simulink model "test_dram_sim"  (Simulink 6.2)
settings: Solver=ode45  StartTime=0.0  StopTime=14000  RelTol=1e-3
undefined symbols (not defined in the file): ant_bits
libraries: xbsIndex_r3 x353, xps_library x9, casper_library x8
(part 1 of 2)
settings Model: LastModifiedBy=humbert
settings DebuggingCC: SolverPrmCheckMsg=warning

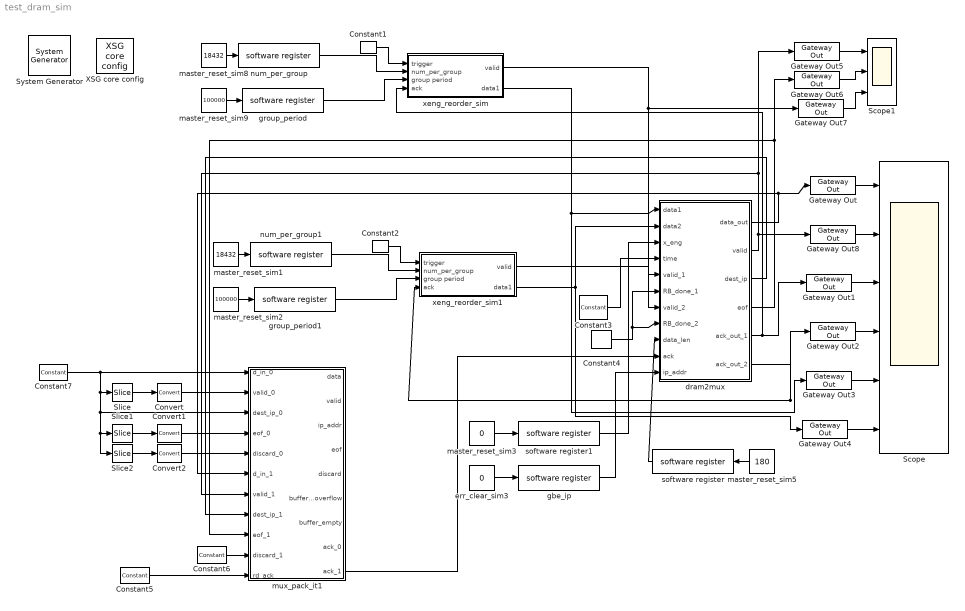
== system test_dram_sim ==
  " System Generator" : xbsIndex_r3/ System Generator  Tag=genX  xilinxfamily=Virtex2  part=xc2v1000  speed=-4  package=bg575  synthesis_tool=XST  directory=./netlist  testbench=off  simulink_period=1  sysclk_period=100  incr_netlist=off  trim_vbits=Everywhere in SubSystem  dbl_ovrd=According to Block Masks  core_generation=According to Block Masks  run_coregen=off  deprecated_control=off  eval_field=0
      settings: AttributesFormatString=System\nGenerator
  Constant1 : xbsIndex_r3/Constant  const=1  equ=P=C  arith_type=Boolean  n_bits=1  bin_pt=0  opselect=C  inp2=PCIN>>17  opr=+  inp1=P  carry=CIN  iostate=0  explicit_period=on  period=1  dbl_ovrd=off
  Constant2 : xbsIndex_r3/Constant  const=1  equ=P=C  arith_type=Boolean  n_bits=1  bin_pt=0  opselect=C  inp2=PCIN>>17  opr=+  inp1=P  carry=CIN  iostate=0  explicit_period=on  period=1  dbl_ovrd=off
  Constant3 : xbsIndex_r3/Constant  const=300  equ=P=C  arith_type=Unsigned  n_bits=64  bin_pt=0  opselect=C  inp2=PCIN>>17  opr=+  inp1=P  carry=CIN  iostate=0  explicit_period=on  period=1  dbl_ovrd=off
  Constant4 : xbsIndex_r3/Constant  const=0  equ=P=C  arith_type=Unsigned  n_bits=1  bin_pt=0  opselect=C  inp2=PCIN>>17  opr=+  inp1=P  carry=CIN  iostate=0  explicit_period=on  period=1  dbl_ovrd=off
  Constant5 : xbsIndex_r3/Constant  const=1  equ=P=C  arith_type=Boolean  n_bits=1  bin_pt=0  opselect=C  inp2=PCIN>>17  opr=+  inp1=P  carry=CIN  iostate=0  explicit_period=on  period=1  dbl_ovrd=off
  Constant6 : xbsIndex_r3/Constant  const=0  equ=P=C  arith_type=Boolean  n_bits=32  bin_pt=0  opselect=C  inp2=PCIN>>17  opr=+  inp1=P  carry=CIN  iostate=0  explicit_period=on  period=1  dbl_ovrd=off
  Constant7 : xbsIndex_r3/Constant  const=0  equ=P=C  arith_type=Unsigned  n_bits=32  bin_pt=0  opselect=C  inp2=PCIN>>17  opr=+  inp1=P  carry=CIN  iostate=0  explicit_period=on  period=1  dbl_ovrd=off
  Convert : xbsIndex_r3/Convert  arith_type=Boolean  n_bits=8  bin_pt=6  quantization=Truncate  overflow=Wrap  latency=0  explicit_period=off  period=1  dbl_ovrd=off  show_param=off  inserted_by_tool=off  pipeline=off
      settings: xl_area=[0, 0, 0, 0, 0, 0, 0]
  Convert1 : xbsIndex_r3/Convert  arith_type=Boolean  n_bits=8  bin_pt=6  quantization=Truncate  overflow=Wrap  latency=0  explicit_period=off  period=1  dbl_ovrd=off  show_param=off  inserted_by_tool=off  pipeline=off
      settings: xl_area=[0, 0, 0, 0, 0, 0, 0]
  Convert2 : xbsIndex_r3/Convert  arith_type=Boolean  n_bits=8  bin_pt=6  quantization=Truncate  overflow=Wrap  latency=0  explicit_period=off  period=1  dbl_ovrd=off  show_param=off  inserted_by_tool=off  pipeline=off
      settings: xl_area=[0, 0, 0, 0, 0, 0, 0]
  Gateway Out{,1..8} (9 alike) : xbsIndex_r3/Gateway Out  output_type=Double  nbits=8  bin_pt=6  arith_type=Boolean  quantization=Truncate  overflow=Wrap  hdl_port=on  timing_constraint=None  locs_specified=off  LOCs={}  needs_fixed_name=off  show_param=off
      settings: xl_area=[0, 0, 0, 0, 0, 0, 0]
  Scope : Scope  NumInputPorts=6
      settings: YMin=0~0~0~0~965~900  YMax=1000~1~1~1~995~930  MaxDataPoints=10000
  Scope1 : Scope  NumInputPorts=3
      settings: YMin=-5~-5~-5  YMax=5~5~5  SaveName=ScopeData6  MaxDataPoints=10000
  Slice : xbsIndex_r3/Slice  mode=Lower Bit Location + Width  nbits=1  bit1=0  base1=MSB of Input  bit0=0  base0=LSB of Input  boolean_output=off  explicit_period=off  period=1  dbl_ovrd=off
  Slice1 : xbsIndex_r3/Slice  mode=Lower Bit Location + Width  nbits=1  bit1=0  base1=MSB of Input  bit0=0  base0=LSB of Input  boolean_output=off  explicit_period=off  period=1  dbl_ovrd=off
  Slice2 : xbsIndex_r3/Slice  mode=Lower Bit Location + Width  nbits=1  bit1=0  base1=MSB of Input  bit0=0  base0=LSB of Input  boolean_output=off  explicit_period=off  period=1  dbl_ovrd=off
  XSG core config : xps_library/XSG core config  Tag=xps:xsg  hw_sys=BEE2_usr  ibob_linux=off  clk_src=sys_clk2x  gpio_clk_io_group=iBOB:sma  gpio_clk_bit_index=0  clk_rate=205  sample_period=1  synthesis_tool=XST  mpc_type=powerpc405
  dram2mux : Subsystem
  err_clear_sim3 : Constant  Value=0
  gbe_ip : xps_library/software register  Tag=xps:sw_reg  io_dir=From Processor  arith_type=Unsigned  bitwidth=32  bin_pt=0  sample_period=1  gw_name=test_dram_sim_gbe_ip_user_data_out
  group_period : xps_library/software register  Tag=xps:sw_reg  io_dir=From Processor  arith_type=Unsigned  bitwidth=32  bin_pt=0  sample_period=1  gw_name=test_dram_sim_group_period_user_data_out
  group_period1 : xps_library/software register  Tag=xps:sw_reg  io_dir=From Processor  arith_type=Unsigned  bitwidth=32  bin_pt=0  sample_period=1  gw_name=test_dram_sim_group_period1_user_data_out
  master_reset_sim1 : Constant  Value=18432
  master_reset_sim2 : Constant  Value=100000
  master_reset_sim3 : Constant  Value=0
  master_reset_sim5 : Constant  Orientation=left  Value=180
  master_reset_sim8 : Constant  Value=18432
  master_reset_sim9 : Constant  Value=100000
  mux_pack_it1 : Subsystem  mask(mux_packets){max_packet_size_0=1500, min_packet_size_0=50, max_packet_size_1=1500, min_packet_size_1=50}
      mask prompts: max_packet_size_0 "Input 0: Maximum single packet size (words)"; min_packet_size_0 "Input 0: Minimum single packet size (words)"; max_packet_size_1 "Input 1: Maximum single packet size (words)"; min_packet_size_1 "Input 1: Minimum single packet size (words)"
      mask help: This block allows you to mux together two data streams to be sent to the 10GbE core
  num_per_group : xps_library/software register  Tag=xps:sw_reg  io_dir=From Processor  arith_type=Unsigned  bitwidth=32  bin_pt=0  sample_period=1  gw_name=test_dram_sim_num_per_group_user_data_out
  num_per_group1 : xps_library/software register  Tag=xps:sw_reg  io_dir=From Processor  arith_type=Unsigned  bitwidth=32  bin_pt=0  sample_period=1  gw_name=test_dram_sim_num_per_group1_user_data_out
  software register : xps_library/software register  Tag=xps:sw_reg  Orientation=left  io_dir=From Processor  arith_type=Unsigned  bitwidth=32  bin_pt=0  sample_period=1  gw_name=test_dram_sim_software_register_user_data_out
  software register1 : xps_library/software register  Tag=xps:sw_reg  io_dir=From Processor  arith_type=Unsigned  bitwidth=32  bin_pt=0  sample_period=1  gw_name=test_dram_sim_software_register1_user_data_out
  xeng_reorder_sim : Subsystem
  xeng_reorder_sim1 : Subsystem
  wires:
  num_per_group/1 -> xeng_reorder_sim/2(num_per_group)
  master_reset_sim8/1 -> num_per_group/1
  group_period/1 -> xeng_reorder_sim/3(group period)
  master_reset_sim9/1 -> group_period/1
  Constant1/1 -> xeng_reorder_sim/1(trigger)
  num_per_group1/1 -> xeng_reorder_sim1/2(num_per_group)
  master_reset_sim1/1 -> num_per_group1/1
  group_period1/1 -> xeng_reorder_sim1/3(group period)
  master_reset_sim2/1 -> group_period1/1
  Constant2/1 -> xeng_reorder_sim1/1(trigger)
  xeng_reorder_sim/2(data1) -> Gateway Out3/1, dram2mux/1(data1)
  xeng_reorder_sim1/2(data1) -> Gateway Out4/1, dram2mux/2(data2)
  xeng_reorder_sim/1(valid) -> dram2mux/5(valid_1), Gateway Out7/1
  xeng_reorder_sim1/1(valid) -> dram2mux/7(valid_2)
  master_reset_sim3/1 -> software register1/1
  software register1/1 -> dram2mux/3(x_eng)
  Constant3/1 -> dram2mux/4(time)
  Constant4/1 -> dram2mux/8(RB_done_2), dram2mux/6(RB_done_1)
  master_reset_sim5/1 -> software register/1
  software register/1 -> dram2mux/9(data_len)
  err_clear_sim3/1 -> gbe_ip/1
  gbe_ip/1 -> dram2mux/11(ip_addr)
  dram2mux/5(ack_out_1) -> xeng_reorder_sim/4(ack), Gateway Out1/1
  dram2mux/6(ack_out_2) -> xeng_reorder_sim1/4(ack), Gateway Out2/1
  Gateway Out/1 -> Scope/1
  dram2mux/1(data_out) -> Gateway Out/1, mux_pack_it1/6(d_in_1)
  dram2mux/2(valid) -> mux_pack_it1/7(valid_1), Gateway Out5/1, Gateway Out8/1
  dram2mux/3(dest_ip) -> mux_pack_it1/8(dest_ip_1)
  Constant5/1 -> mux_pack_it1/11(rd_ack)
  Constant6/1 -> mux_pack_it1/10(discard_1)
  mux_pack_it1/9(ack_1) -> dram2mux/10(ack)
  Constant7/1 -> mux_pack_it1/1(d_in_0), mux_pack_it1/3(dest_ip_0), Slice1/1, Slice2/1, Slice/1
  Slice/1 -> Convert/1
  Convert/1 -> mux_pack_it1/2(valid_0)
  Slice1/1 -> Convert1/1
  Slice2/1 -> Convert2/1
  Convert1/1 -> mux_pack_it1/4(eof_0)
  Convert2/1 -> mux_pack_it1/5(discard_0)
  Gateway Out5/1 -> Scope1/1
  Gateway Out6/1 -> Scope1/2
  dram2mux/4(eof) -> mux_pack_it1/9(eof_1), Gateway Out6/1
  Gateway Out7/1 -> Scope1/3
  Gateway Out4/1 -> Scope/6
  Gateway Out3/1 -> Scope/5
  Gateway Out2/1 -> Scope/4
  Gateway Out1/1 -> Scope/3
  Gateway Out8/1 -> Scope/2

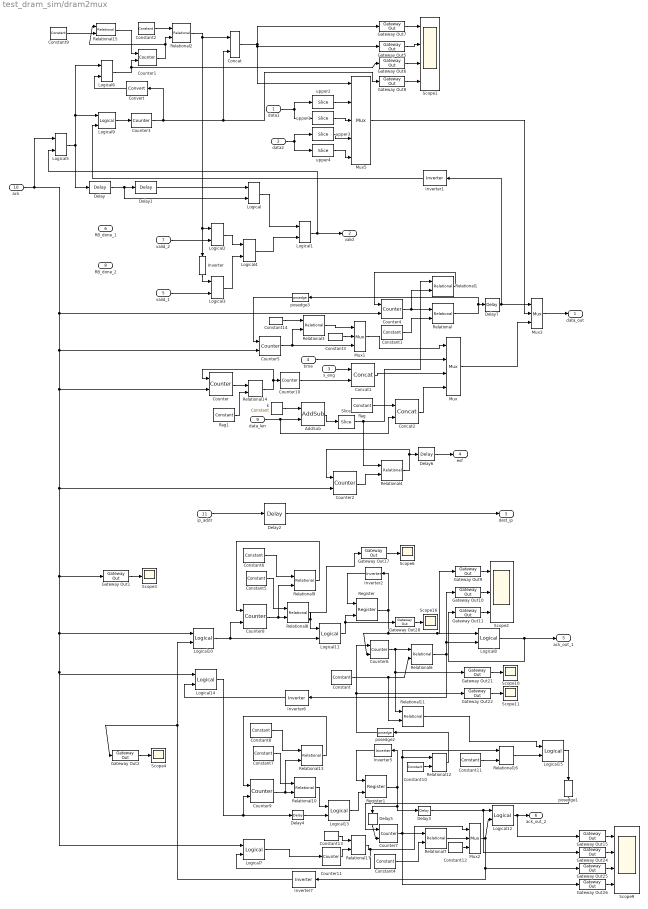
== system test_dram_sim/dram2mux ==
  data1 : Inport  Port=1  LatchInput=off
  data2 : Inport  Port=2  LatchInput=off
  x_eng : Inport  Port=3  LatchInput=off
  time : Inport  Port=4  LatchInput=off
  valid_1 : Inport  Port=5  LatchInput=off
  RB_done_1 : Inport  Port=6  LatchInput=off
  valid_2 : Inport  Port=7  LatchInput=off
  RB_done_2 : Inport  Port=8  LatchInput=off
  data_len : Inport  Port=9  LatchInput=off
  ack : Inport  Port=10  LatchInput=off
  ip_addr : Inport  Port=11  LatchInput=off
  AddSub : xbsIndex_r3/AddSub  mode=Addition  precision=Full  arith_type=Unsigned  n_bits=8  bin_pt=2  quantization=Truncate  overflow=Wrap  latency=0  explicit_period=off  period=1  use_carryin=off  use_carryout=off  en=off  dbl_ovrd=off  show_param=off  use_core=on  pipeline=off  use_rpm=on  gen_core=off
      settings: xl_area=[0, 0, 0, 0, 0, 0, 0]
  Concat : xbsIndex_r3/Concat  num_inputs=2  explicit_period=off  period=1  dbl_ovrd=off
  Concat1 : xbsIndex_r3/Concat  num_inputs=2  explicit_period=off  period=1  dbl_ovrd=off
  Concat2 : xbsIndex_r3/Concat  num_inputs=2  explicit_period=off  period=1  dbl_ovrd=off
  Constant : xbsIndex_r3/Constant  const=269  equ=P=C  arith_type=Unsigned  n_bits=9  bin_pt=0  opselect=C  inp2=PCIN>>17  opr=+  inp1=P  carry=CIN  iostate=0  explicit_period=on  period=1  dbl_ovrd=off
  Constant1 : xbsIndex_r3/Constant  const=3  equ=P=C  arith_type=Unsigned  n_bits=16  bin_pt=0  opselect=C  inp2=PCIN>>17  opr=+  inp1=P  carry=CIN  iostate=0  explicit_period=on  period=1  dbl_ovrd=off
  Constant10 : xbsIndex_r3/Constant  const=269  equ=P=C  arith_type=Unsigned  n_bits=9  bin_pt=0  opselect=C  inp2=PCIN>>17  opr=+  inp1=P  carry=CIN  iostate=0  explicit_period=on  period=1  dbl_ovrd=off
  Constant11 : xbsIndex_r3/Constant  const=271  equ=P=C  arith_type=Unsigned  n_bits=9  bin_pt=0  opselect=C  inp2=PCIN>>17  opr=+  inp1=P  carry=CIN  iostate=0  explicit_period=on  period=1  dbl_ovrd=off
  Constant12 : xbsIndex_r3/Constant  const=0  equ=P=C  arith_type=Boolean  n_bits=1  bin_pt=0  opselect=C  inp2=PCIN>>17  opr=+  inp1=P  carry=CIN  iostate=0  explicit_period=on  period=1  dbl_ovrd=off
  Constant13 : xbsIndex_r3/Constant  const=183  equ=P=C  arith_type=Unsigned  n_bits=10  bin_pt=0  opselect=C  inp2=PCIN>>17  opr=+  inp1=P  carry=CIN  iostate=0  explicit_period=on  period=1  dbl_ovrd=off
  Constant14 : xbsIndex_r3/Constant  const=2  equ=P=C  arith_type=Unsigned  n_bits=2  bin_pt=0  opselect=C  inp2=PCIN>>17  opr=+  inp1=P  carry=CIN  iostate=0  explicit_period=on  period=1  dbl_ovrd=off
  Constant2 : xbsIndex_r3/Constant  const=90  equ=P=C  arith_type=Unsigned  n_bits=8  bin_pt=0  opselect=C  inp2=PCIN>>17  opr=+  inp1=P  carry=CIN  iostate=0  explicit_period=on  period=1  dbl_ovrd=off
  Constant3 : xbsIndex_r3/Constant  const=0  equ=P=C  arith_type=Unsigned  n_bits=1  bin_pt=0  opselect=C  inp2=PCIN>>17  opr=+  inp1=P  carry=CIN  iostate=0  explicit_period=on  period=1  dbl_ovrd=off
  Constant4 : xbsIndex_r3/Constant  const=269  equ=P=C  arith_type=Unsigned  n_bits=9  bin_pt=0  opselect=C  inp2=PCIN>>17  opr=+  inp1=P  carry=CIN  iostate=0  explicit_period=on  period=1  dbl_ovrd=off
  Constant5 : xbsIndex_r3/Constant  const=3  equ=P=C  arith_type=Unsigned  n_bits=2  bin_pt=0  opselect=C  inp2=PCIN>>17  opr=+  inp1=P  carry=CIN  iostate=0  explicit_period=on  period=1  dbl_ovrd=off
  Constant6 : xbsIndex_r3/Constant  const=183  equ=P=C  arith_type=Unsigned  n_bits=8  bin_pt=0  opselect=C  inp2=PCIN>>17  opr=+  inp1=P  carry=CIN  iostate=0  explicit_period=on  period=1  dbl_ovrd=off
  Constant7 : xbsIndex_r3/Constant  const=3  equ=P=C  arith_type=Unsigned  n_bits=2  bin_pt=0  opselect=C  inp2=PCIN>>17  opr=+  inp1=P  carry=CIN  iostate=0  explicit_period=on  period=1  dbl_ovrd=off
  Constant8 : xbsIndex_r3/Constant  const=183  equ=P=C  arith_type=Unsigned  n_bits=8  bin_pt=0  opselect=C  inp2=PCIN>>17  opr=+  inp1=P  carry=CIN  iostate=0  explicit_period=on  period=1  dbl_ovrd=off
  Constant9 : xbsIndex_r3/Constant  const=180  equ=P=C  arith_type=Unsigned  n_bits=8  bin_pt=0  opselect=C  inp2=PCIN>>17  opr=+  inp1=P  carry=CIN  iostate=0  explicit_period=on  period=1  dbl_ovrd=off
  Convert : xbsIndex_r3/Convert  Orientation=left  arith_type=Boolean  n_bits=8  bin_pt=6  quantization=Truncate  overflow=Wrap  latency=0  explicit_period=off  period=1  dbl_ovrd=off  show_param=off  inserted_by_tool=off  pipeline=off
      settings: xl_area=[0, 0, 0, 0, 0, 0, 0]
  Counter : xbsIndex_r3/Counter  cnt_type=Free Running  n_bits=32  bin_pt=0  arith_type=Unsigned  start_count=0  cnt_to=Inf  cnt_by_val=1  operation=Up  explicit_period=on  period=1  load_pin=off  rst=on  en=on  dbl_ovrd=off  show_param=off  use_rpm=on  gen_core=off
      settings: xl_area=[0, 0, 0, 0, 0, 0, 0]
  Counter1 : xbsIndex_r3/Counter  cnt_type=Free Running  n_bits=8  bin_pt=0  arith_type=Unsigned  start_count=0  cnt_to=180  cnt_by_val=1  operation=Up  explicit_period=on  period=1  load_pin=off  rst=on  en=on  dbl_ovrd=off  show_param=off  use_rpm=on  gen_core=off
      settings: xl_area=[0, 0, 0, 0, 0, 0, 0]
  Counter10 : xbsIndex_r3/Counter  cnt_type=Free Running  n_bits=32  bin_pt=0  arith_type=Unsigned  start_count=0  cnt_to=Inf  cnt_by_val=1  operation=Up  explicit_period=on  period=1  load_pin=off  rst=off  en=on  dbl_ovrd=off  show_param=off  use_rpm=on  gen_core=off
      settings: xl_area=[0, 0, 0, 0, 0, 0, 0]
  Counter11 : xbsIndex_r3/Counter  cnt_type=Free Running  n_bits=10  bin_pt=0  arith_type=Unsigned  start_count=0  cnt_to=Inf  cnt_by_val=1  operation=Up  explicit_period=on  period=1  load_pin=off  rst=off  en=on  dbl_ovrd=off  show_param=off  use_rpm=on  gen_core=off
      settings: xl_area=[0, 0, 0, 0, 0, 0, 0]
  Counter2 : xbsIndex_r3/Counter  cnt_type=Free Running  n_bits=32  bin_pt=0  arith_type=Unsigned  start_count=0  cnt_to=Inf  cnt_by_val=1  operation=Up  explicit_period=on  period=1  load_pin=off  rst=on  en=on  dbl_ovrd=off  show_param=off  use_rpm=on  gen_core=off
      settings: xl_area=[0, 0, 0, 0, 0, 0, 0]
  Counter3 : xbsIndex_r3/Counter  cnt_type=Free Running  n_bits=1  bin_pt=0  arith_type=Unsigned  start_count=0  cnt_to=Inf  cnt_by_val=1  operation=Up  explicit_period=on  period=1  load_pin=off  rst=off  en=on  dbl_ovrd=off  show_param=off  use_rpm=on  gen_core=off
      settings: xl_area=[0, 0, 0, 0, 0, 0, 0]
  Counter4 : xbsIndex_r3/Counter  cnt_type=Free Running  n_bits=16  bin_pt=0  arith_type=Unsigned  start_count=0  cnt_to=Inf  cnt_by_val=1  operation=Up  explicit_period=on  period=1  load_pin=off  rst=on  en=on  dbl_ovrd=off  show_param=off  use_rpm=on  gen_core=off
      settings: xl_area=[0, 0, 0, 0, 0, 0, 0]
  Counter5 : xbsIndex_r3/Counter  cnt_type=Free Running  n_bits=2  bin_pt=0  arith_type=Unsigned  start_count=0  cnt_to=Inf  cnt_by_val=1  operation=Up  explicit_period=on  period=1  load_pin=off  rst=on  en=on  dbl_ovrd=off  show_param=off  use_rpm=on  gen_core=off
      settings: xl_area=[0, 0, 0, 0, 0, 0, 0]
  Counter6 : xbsIndex_r3/Counter  cnt_type=Free Running  n_bits=10  bin_pt=0  arith_type=Unsigned  start_count=0  cnt_to=Inf  cnt_by_val=1  operation=Up  explicit_period=on  period=1  load_pin=off  rst=on  en=on  dbl_ovrd=off  show_param=off  use_rpm=on  gen_core=off
      settings: xl_area=[0, 0, 0, 0, 0, 0, 0]
  Counter7 : xbsIndex_r3/Counter  cnt_type=Free Running  n_bits=10  bin_pt=0  arith_type=Unsigned  start_count=0  cnt_to=Inf  cnt_by_val=1  operation=Up  explicit_period=on  period=1  load_pin=off  rst=on  en=on  dbl_ovrd=off  show_param=off  use_rpm=on  gen_core=off
      settings: xl_area=[0, 0, 0, 0, 0, 0, 0]
  Counter8 : xbsIndex_r3/Counter  cnt_type=Free Running  n_bits=8  bin_pt=0  arith_type=Unsigned  start_count=0  cnt_to=Inf  cnt_by_val=1  operation=Up  explicit_period=on  period=1  load_pin=off  rst=on  en=on  dbl_ovrd=off  show_param=off  use_rpm=on  gen_core=off
      settings: xl_area=[0, 0, 0, 0, 0, 0, 0]
  Counter9 : xbsIndex_r3/Counter  cnt_type=Free Running  n_bits=8  bin_pt=0  arith_type=Unsigned  start_count=0  cnt_to=Inf  cnt_by_val=1  operation=Up  explicit_period=on  period=1  load_pin=off  rst=on  en=on  dbl_ovrd=off  show_param=off  use_rpm=on  gen_core=off
      settings: xl_area=[0, 0, 0, 0, 0, 0, 0]
  Delay : xbsIndex_r3/Delay  latency=1  reg_retiming=off  explicit_period=on  period=1  en=off  accept_only_valid=off  init_zero=on  dbl_ovrd=off  show_param=off
      settings: xl_area=[0, 0, 0, 0, 0, 0, 0]
  Delay1 : xbsIndex_r3/Delay  latency=1  reg_retiming=off  explicit_period=on  period=1  en=off  accept_only_valid=off  init_zero=on  dbl_ovrd=off  show_param=off
      settings: xl_area=[0, 0, 0, 0, 0, 0, 0]
  Delay2 : xbsIndex_r3/Delay  latency=2  reg_retiming=off  explicit_period=off  period=1  en=off  accept_only_valid=off  init_zero=on  dbl_ovrd=off  show_param=off
      settings: xl_area=[0, 0, 0, 0, 0, 0, 0]
  Delay3 : xbsIndex_r3/Delay  latency=1  reg_retiming=off  explicit_period=on  period=1  en=off  accept_only_valid=off  init_zero=on  dbl_ovrd=off  show_param=off
      settings: xl_area=[0, 0, 0, 0, 0, 0, 0]
  Delay4 : xbsIndex_r3/Delay  latency=2  reg_retiming=off  explicit_period=on  period=1  en=off  accept_only_valid=off  init_zero=on  dbl_ovrd=off  show_param=off
      settings: xl_area=[0, 0, 0, 0, 0, 0, 0]
  Delay5 : xbsIndex_r3/Delay  Orientation=down  latency=1  reg_retiming=off  explicit_period=on  period=1  en=off  accept_only_valid=off  init_zero=on  dbl_ovrd=off  show_param=off
      settings: xl_area=[0, 0, 0, 0, 0, 0, 0]
  Delay6 : xbsIndex_r3/Delay  latency=1  reg_retiming=off  explicit_period=off  period=1  en=off  accept_only_valid=off  init_zero=on  dbl_ovrd=off  show_param=off
      settings: xl_area=[0, 0, 0, 0, 0, 0, 0]
  Delay7 : xbsIndex_r3/Delay  latency=1  reg_retiming=off  explicit_period=off  period=1  en=off  accept_only_valid=off  init_zero=on  dbl_ovrd=off  show_param=off
      settings: xl_area=[0, 0, 0, 0, 0, 0, 0]
  Gateway Out{1..2,5..11,15,17,21..22,24..26,28} (17 alike) : xbsIndex_r3/Gateway Out  output_type=Double  nbits=8  bin_pt=6  arith_type=Boolean  quantization=Truncate  overflow=Wrap  hdl_port=on  timing_constraint=None  locs_specified=off  LOCs={}  needs_fixed_name=off  show_param=off
      settings: xl_area=[0, 0, 0, 0, 0, 0, 0]
  Inverter : xbsIndex_r3/Inverter  Orientation=down  latency=0  explicit_period=off  period=1  en=off  dbl_ovrd=off  show_param=off
      settings: xl_area=[0, 0, 0, 0, 0, 0, 0]
  Inverter{1..2,5..7} (5 alike) : xbsIndex_r3/Inverter  Orientation=left  latency=0  explicit_period=off  period=1  en=off  dbl_ovrd=off  show_param=off
      settings: xl_area=[0, 0, 0, 0, 0, 0, 0]
  Logical : xbsIndex_r3/Logical  logical_function=NOR  inputs=2  precision=Full  arith_type=Unsigned  n_bits=8  bin_pt=2  align_bp=on  latency=0  explicit_period=off  period=1  en=off  dbl_ovrd=off  show_param=off
      settings: xl_area=[0, 0, 0, 0, 0, 0, 0]
  Logical{1..3,5..6} (5 alike) : xbsIndex_r3/Logical  logical_function=AND  inputs=2  precision=Full  arith_type=Unsigned  n_bits=8  bin_pt=2  align_bp=off  latency=0  explicit_period=off  period=1  en=off  dbl_ovrd=off  show_param=off
      settings: xl_area=[0, 0, 0, 0, 0, 0, 0]
  Logical{7,9..11,13..14} (6 alike) : xbsIndex_r3/Logical  logical_function=AND  inputs=2  precision=Full  arith_type=Unsigned  n_bits=8  bin_pt=2  align_bp=on  latency=0  explicit_period=off  period=1  en=off  dbl_ovrd=off  show_param=off
      settings: xl_area=[0, 0, 0, 0, 0, 0, 0]
  Logical12 : xbsIndex_r3/Logical  logical_function=AND  inputs=2  precision=Full  arith_type=Unsigned  n_bits=8  bin_pt=2  align_bp=on  latency=2  explicit_period=on  period=1  en=off  dbl_ovrd=off  show_param=off
      settings: xl_area=[0, 0, 0, 0, 0, 0, 0]
  Logical15 : xbsIndex_r3/Logical  logical_function=OR  inputs=2  precision=Full  arith_type=Unsigned  n_bits=8  bin_pt=2  align_bp=on  latency=0  explicit_period=off  period=1  en=off  dbl_ovrd=off  show_param=off
      settings: xl_area=[0, 0, 0, 0, 0, 0, 0]
  Logical4 : xbsIndex_r3/Logical  logical_function=OR  inputs=2  precision=Full  arith_type=Unsigned  n_bits=8  bin_pt=2  align_bp=on  latency=2  explicit_period=off  period=1  en=off  dbl_ovrd=off  show_param=off
      settings: xl_area=[0, 0, 0, 0, 0, 0, 0]
  Logical8 : xbsIndex_r3/Logical  logical_function=AND  inputs=2  precision=Full  arith_type=Unsigned  n_bits=8  bin_pt=2  align_bp=on  latency=2  explicit_period=on  period=1  en=off  dbl_ovrd=off  show_param=off
      settings: xl_area=[0, 0, 0, 0, 0, 0, 0]
  Mux : xbsIndex_r3/Mux  inputs=3  precision=Full  arith_type="Signed  (2's comp)"  n_bits=8  bin_pt=2  quantization=Truncate  overflow=Wrap  latency=2  explicit_period=on  period=1  en=off  dbl_ovrd=off  show_param=off  mux_type=off  use_rpm=off  gen_core=off
      settings: xl_area=[0, 0, 0, 0, 0, 0, 0]
  Mux1 : xbsIndex_r3/Mux  inputs=2  precision=Full  arith_type="Signed  (2's comp)"  n_bits=8  bin_pt=2  quantization=Truncate  overflow=Wrap  latency=0  explicit_period=off  period=1  en=off  dbl_ovrd=off  show_param=off  mux_type=off  use_rpm=off  gen_core=off
      settings: xl_area=[0, 0, 0, 0, 0, 0, 0]
  Mux2 : xbsIndex_r3/Mux  inputs=2  precision=Full  arith_type="Signed  (2's comp)"  n_bits=8  bin_pt=2  quantization=Truncate  overflow=Wrap  latency=0  explicit_period=off  period=1  en=off  dbl_ovrd=off  show_param=off  mux_type=off  use_rpm=off  gen_core=off
      settings: xl_area=[0, 0, 0, 0, 0, 0, 0]
  Mux3 : xbsIndex_r3/Mux  inputs=2  precision=Full  arith_type="Signed  (2's comp)"  n_bits=8  bin_pt=2  quantization=Truncate  overflow=Wrap  latency=0  explicit_period=off  period=1  en=off  dbl_ovrd=off  show_param=off  mux_type=off  use_rpm=off  gen_core=off
      settings: xl_area=[0, 0, 0, 0, 0, 0, 0]
  Mux5 : xbsIndex_r3/Mux  inputs=4  precision=Full  arith_type="Signed  (2's comp)"  n_bits=8  bin_pt=2  quantization=Truncate  overflow=Wrap  latency=2  explicit_period=on  period=1  en=off  dbl_ovrd=off  show_param=off  mux_type=off  use_rpm=off  gen_core=off
      settings: xl_area=[0, 0, 0, 0, 0, 0, 0]
  Register : xbsIndex_r3/Register  init=0  reg_only_valid=off  explicit_period=on  period=1  rst=off  en=on  out_en=off  dbl_ovrd=off  show_param=off
      settings: xl_area=[0, 0, 0, 0, 0, 0, 0]
  Register1 : xbsIndex_r3/Register  init=0  reg_only_valid=off  explicit_period=on  period=1  rst=off  en=on  out_en=off  dbl_ovrd=off  show_param=off
      settings: xl_area=[0, 0, 0, 0, 0, 0, 0]
  Relational : xbsIndex_r3/Relational  mode=a<b  latency=0  explicit_period=off  period=1  en=off  dbl_ovrd=off  show_param=off
      settings: xl_area=[0, 0, 0, 0, 0, 0, 0]
  Relational{1,4,9,12..14,16} (7 alike) : xbsIndex_r3/Relational  mode=a=b  latency=0  explicit_period=off  period=1  en=off  dbl_ovrd=off  show_param=off
      settings: xl_area=[0, 0, 0, 0, 0, 0, 0]
  Relational{2,6..8,10} (5 alike) : xbsIndex_r3/Relational  mode=a<=b  latency=0  explicit_period=off  period=1  en=off  dbl_ovrd=off  show_param=off
      settings: xl_area=[0, 0, 0, 0, 0, 0, 0]
  Relational11 : xbsIndex_r3/Relational  mode=a=b  latency=0  explicit_period=on  period=1  en=off  dbl_ovrd=off  show_param=off
      settings: xl_area=[0, 0, 0, 0, 0, 0, 0]
  Relational15 : xbsIndex_r3/Relational  mode=a=b  latency=1  explicit_period=off  period=1  en=off  dbl_ovrd=off  show_param=off
      settings: xl_area=[0, 0, 0, 0, 0, 0, 0]
  Relational17 : xbsIndex_r3/Relational  mode=a>b  latency=0  explicit_period=off  period=1  en=off  dbl_ovrd=off  show_param=off
      settings: xl_area=[0, 0, 0, 0, 0, 0, 0]
  Relational3 : xbsIndex_r3/Relational  mode=a>=b  latency=0  explicit_period=off  period=1  en=off  dbl_ovrd=off  show_param=off
      settings: xl_area=[0, 0, 0, 0, 0, 0, 0]
  Scope1 : Scope  NumInputPorts=4
      settings: TimeRange=139.0728476821191  YMin=0~0~0~0  YMax=3~1~1~1  SaveName=ScopeData2
  Scope{3..4,6,10..11,16} (6 alike) : Scope
      Scope10 settings: SaveName=ScopeData16
      Scope11 settings: SaveName=ScopeData17
      Scope16 settings: SaveName=ScopeData22
      Scope3 settings: SaveName=ScopeData7
      Scope4 settings: SaveName=ScopeData8
      Scope6 settings: SaveName=ScopeData12
  Scope2 : Scope  NumInputPorts=3
      settings: TimeRange=1.513091531073314  YMin=0~0~0  YMax=1~1~1  SaveName=ScopeData4
  Scope9 : Scope  NumInputPorts=4
      settings: TimeRange=3000  YMin=-5~-5~-5~-5  YMax=5~5~5~5  SaveName=ScopeData15
  Slice : xbsIndex_r3/Slice  mode=Lower Bit Location + Width  nbits=32  bit1=0  base1=MSB of Input  bit0=0  base0=LSB of Input  boolean_output=off  explicit_period=off  period=1  dbl_ovrd=off
  flag : xbsIndex_r3/Constant  const=0  equ=P=C  arith_type=Unsigned  n_bits=32  bin_pt=0  opselect=C  inp2=PCIN>>17  opr=+  inp1=P  carry=CIN  iostate=0  explicit_period=on  period=1  dbl_ovrd=off
  flag1 : xbsIndex_r3/Constant  const=180  equ=P=C  arith_type=Unsigned  n_bits=32  bin_pt=0  opselect=C  inp2=PCIN>>17  opr=+  inp1=P  carry=CIN  iostate=0  explicit_period=on  period=1  dbl_ovrd=off
  k : xbsIndex_r3/Constant  const=3  equ=P=C  arith_type=Unsigned  n_bits=32  bin_pt=0  opselect=C  inp2=PCIN>>17  opr=+  inp1=P  carry=CIN  iostate=0  explicit_period=on  period=1  dbl_ovrd=off
  posedge1 : casper_library/Misc/posedge  Tag=Rising Edge Detector  Orientation=down
  posedge2 : casper_library/Misc/posedge  Tag=Rising Edge Detector  Orientation=left
  posedge3 : casper_library/Misc/posedge  Tag=Rising Edge Detector  Orientation=left
  upper1 : xbsIndex_r3/Slice  mode=Lower Bit Location + Width  nbits=64  bit1=0  base1=MSB of Input  bit0=0  base0=LSB of Input  boolean_output=off  explicit_period=off  period=1  dbl_ovrd=off
  upper2 : xbsIndex_r3/Slice  mode=Upper Bit Location + Width  nbits=64  bit1=0  base1=MSB of Input  bit0=0  base0=LSB of Input  boolean_output=off  explicit_period=off  period=1  dbl_ovrd=off
  upper3 : xbsIndex_r3/Slice  mode=Upper Bit Location + Width  nbits=64  bit1=0  base1=MSB of Input  bit0=0  base0=LSB of Input  boolean_output=off  explicit_period=off  period=1  dbl_ovrd=off
  upper4 : xbsIndex_r3/Slice  mode=Lower Bit Location + Width  nbits=64  bit1=0  base1=MSB of Input  bit0=0  base0=LSB of Input  boolean_output=off  explicit_period=off  period=1  dbl_ovrd=off
  data_out : Outport
  valid : Outport  Port=2
  dest_ip : Outport  Port=3
  eof : Outport  Port=4
  ack_out_1 : Outport  Port=5
  ack_out_2 : Outport  Port=6
  wires:
  Inverter7/1 -> Logical10/2, Gateway Out2/1
  Logical14/1 -> Counter9/2, Delay4/1
  Inverter6/1 -> Logical14/2
  Logical10/1 -> Counter8/2, Logical11/2
  Logical13/1 -> Register1/2
  Logical12/1 -> ack_out_2/1, Gateway Out15/1
  Constant4/1 -> Relational7/2
  Counter7/1 -> Relational7/1, Gateway Out26/1, Relational12/1, Relational16/1
  Inverter5/1 -> Register1/1
  Register1/1 -> Inverter5/1, Delay3/1, Delay5/1
  Relational9/1 -> Counter8/1
  Constant6/1 -> Relational9/1
  Constant5/1 -> Relational8/1
  Counter8/1 -> Relational8/2, Relational9/2
  Logical8/1 -> ack_out_1/1, Gateway Out11/1
  Relational6/1 -> Inverter6/1, Gateway Out10/1, Logical8/2
  Constant/1 -> Relational6/2, Relational11/2
  Counter6/1 -> Relational6/1, Relational11/1, Gateway Out21/1
  Inverter2/1 -> Register/1
  Register/1 -> Inverter2/1, Counter6/2, Gateway Out9/1, Logical8/1
  Inverter1/1 -> Logical9/2
  Mux5/1 -> Mux3/2
  AddSub/1 -> Slice/1
  k/1 -> AddSub/1
  data_len/1 -> Concat2/2, AddSub/2
  Delay2/1 -> dest_ip/1
  Relational4/1 -> Counter2/1, Delay6/1
  Counter2/1 -> Relational4/2
  ip_addr/1 -> Delay2/1
  Mux3/1 -> data_out/1
  Relational1/1 -> Counter4/1
  Constant1/1 -> Relational/2
  Relational/1 -> posedge3/1, Delay7/1
  Counter4/1 -> Relational/1, Relational1/2
  Mux/1 -> Mux3/3
  flag/1 -> Concat2/1
  x_eng/1 -> Concat1/1
  time/1 -> Mux/2
  Concat1/1 -> Mux/3
  Concat2/1 -> Mux/4
  Logical6/1 -> Gateway Out6/1, Counter1/2
  Logical5/1 -> Logical6/1, Logical9/1, Delay/1
  Logical4/1 -> Logical1/2
  Logical3/1 -> Logical4/2
  Logical2/1 -> Logical4/1
  valid_2/1 -> Logical2/2
  valid_1/1 -> Logical3/2
  Logical1/1 -> valid/1, Logical5/2
  Logical/1 -> Logical1/1
  Delay1/1 -> Logical/1
  Delay/1 -> Delay1/1, Logical/2
  ack/1 -> Logical5/1, Counter2/2, Logical10/1, Logical14/1, Logical7/1, Gateway Out1/1, Counter/2, Counter5/2, Counter4/2
  Concat/1 -> Gateway Out7/1, Mux5/1, Gateway Out5/1
  Relational2/1 -> Concat/1, Logical2/1, Inverter/1
  Counter1/1 -> Relational2/2, Relational15/1
  Constant2/1 -> Relational2/1
  data2/1 -> upper3/1, upper4/1
  data1/1 -> upper2/1, upper1/1
  upper4/1 -> Mux5/5
  upper3/1 -> Mux5/4
  upper1/1 -> Mux5/3
  upper2/1 -> Mux5/2
  Inverter/1 -> Logical3/1
  Convert/1 -> Logical6/2
  Counter/1 -> Relational14/1
  flag1/1 -> Relational14/2
  Relational14/1 -> Counter10/1, Counter/1
  Slice/1 -> Relational4/1, Relational1/1
  Gateway Out7/1 -> Scope1/1
  Gateway Out5/1 -> Scope1/2
  Gateway Out6/1 -> Scope1/3
  Gateway Out8/1 -> Scope1/4
  Counter10/1 -> Concat1/2
  Gateway Out9/1 -> Scope2/1
  Gateway Out10/1 -> Scope2/2
  Gateway Out11/1 -> Scope2/3
  Relational8/1 -> Logical11/1, Gateway Out17/1
  Logical11/1 -> Register/2, Gateway Out28/1
  Counter3/1 -> Convert/1, Gateway Out8/1, Concat/2
  Logical9/1 -> Counter3/1
  Gateway Out17/1 -> Scope6/1
  Relational15/1 -> Counter1/1
  Constant9/1 -> Relational15/2
  Gateway Out21/1 -> Scope10/1
  Gateway Out22/1 -> Scope11/1
  Gateway Out28/1 -> Scope16/1
  Relational13/1 -> Counter9/1
  Constant8/1 -> Relational13/1
  Constant7/1 -> Relational10/1
  Counter9/1 -> Relational10/2, Relational13/2
  Relational10/1 -> Logical13/1
  Delay4/1 -> Logical13/2
  Relational12/1 -> posedge2/1
  Relational11/1 -> Logical15/1
  Constant11/1 -> Relational16/2
  Relational16/1 -> Logical15/2
  posedge1/1 -> Counter7/1
  Logical15/1 -> posedge1/1
  Constant10/1 -> Relational12/2
  posedge2/1 -> Counter6/1, Gateway Out22/1
  Delay3/1 -> Logical12/1, Gateway Out24/1
  Gateway Out15/1 -> Scope9/1
  Gateway Out24/1 -> Scope9/2
  Gateway Out25/1 -> Scope9/3
  Gateway Out26/1 -> Scope9/4
  Mux2/1 -> Logical12/2, Inverter7/1, Gateway Out25/1
  Relational7/1 -> Mux2/2
  Constant12/1 -> Mux2/3
  Constant13/1 -> Relational17/1
  Counter11/1 -> Relational17/2
  Relational17/1 -> Mux2/1, Logical7/2
  Delay5/1 -> Counter7/2
  Delay6/1 -> eof/1
  Delay7/1 -> Inverter1/1, Mux3/1
  posedge3/1 -> Counter5/1
  Mux1/1 -> Mux/1
  Counter5/1 -> Mux1/3, Relational3/2
  Constant3/1 -> Mux1/2
  Constant14/1 -> Relational3/1
  Relational3/1 -> Mux1/1
  Logical7/1 -> Counter11/1
  Gateway Out1/1 -> Scope3/1
  Gateway Out2/1 -> Scope4/1

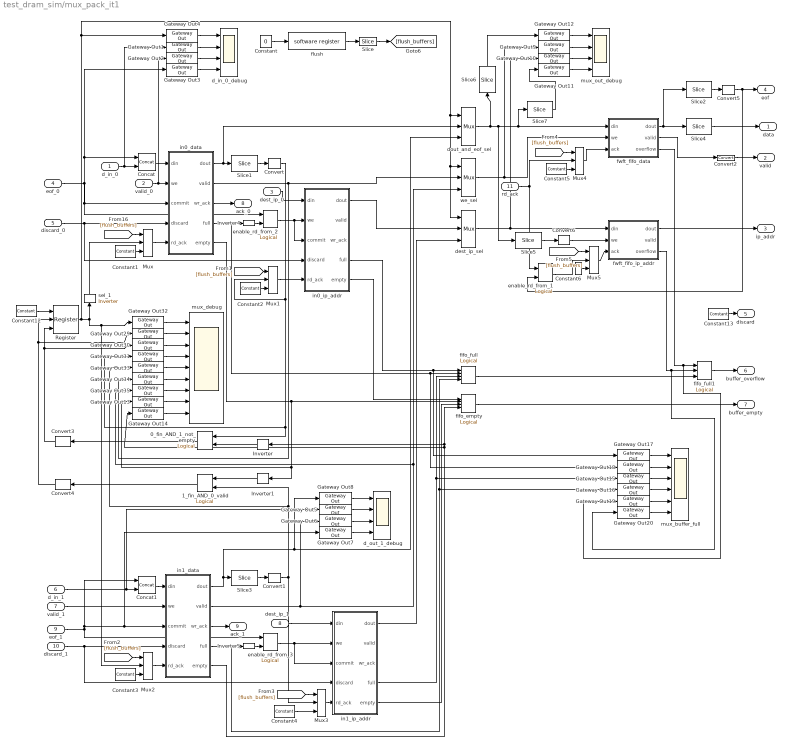
== system test_dram_sim/mux_pack_it1 ==
  d_in_0 : Inport  Port=1  LatchInput=off
  valid_0 : Inport  Port=2  LatchInput=off
  dest_ip_0 : Inport  Port=3  LatchInput=off
  eof_0 : Inport  Port=4  LatchInput=off
  discard_0 : Inport  Port=5  LatchInput=off
  d_in_1 : Inport  Port=6  LatchInput=off
  valid_1 : Inport  Port=7  LatchInput=off
  dest_ip_1 : Inport  Port=8  LatchInput=off
  eof_1 : Inport  Port=9  LatchInput=off
  discard_1 : Inport  Port=10  LatchInput=off
  rd_ack : Inport  Port=11  LatchInput=off
  0_fin_AND_1_not_empty : xbsIndex_r3/Logical  Orientation=left  logical_function=AND  inputs=2  precision=Full  arith_type=Unsigned  n_bits=8  bin_pt=2  align_bp=on  latency=0  explicit_period=on  period=1  en=off  dbl_ovrd=off  show_param=off
      settings: xl_area=[0, 0, 0, 0, 0, 0, 0]
  1_fin_AND_0_valid : xbsIndex_r3/Logical  Orientation=left  logical_function=AND  inputs=2  precision=Full  arith_type=Unsigned  n_bits=8  bin_pt=2  align_bp=on  latency=0  explicit_period=on  period=1  en=off  dbl_ovrd=off  show_param=off
      settings: xl_area=[0, 0, 0, 0, 0, 0, 0]
  Concat : xbsIndex_r3/Concat  num_inputs=2  explicit_period=off  period=1  dbl_ovrd=off
  Concat1 : xbsIndex_r3/Concat  num_inputs=2  explicit_period=off  period=1  dbl_ovrd=off
  Constant : Constant  Value=0
  Constant{1..6,12} (7 alike) : xbsIndex_r3/Constant  const=1  equ=P=C  arith_type=Boolean  n_bits=1  bin_pt=0  opselect=C  inp2=PCIN>>17  opr=+  inp1=P  carry=CIN  iostate=0  explicit_period=on  period=1  dbl_ovrd=off
  Constant13 : xbsIndex_r3/Constant  const=0  equ=P=C  arith_type=Boolean  n_bits=1  bin_pt=0  opselect=C  inp2=PCIN>>17  opr=+  inp1=P  carry=CIN  iostate=0  explicit_period=on  period=1  dbl_ovrd=off
  Convert{,1..2,5..6} (5 alike) : xbsIndex_r3/Convert  arith_type=Boolean  n_bits=8  bin_pt=6  quantization=Truncate  overflow=Wrap  latency=0  explicit_period=off  period=1  dbl_ovrd=off  show_param=off  inserted_by_tool=off  pipeline=off
      settings: xl_area=[0, 0, 0, 0, 0, 0, 0]
  Convert3 : xbsIndex_r3/Convert  Orientation=left  arith_type=Boolean  n_bits=8  bin_pt=6  quantization=Truncate  overflow=Wrap  latency=0  explicit_period=off  period=1  dbl_ovrd=off  show_param=off  inserted_by_tool=off  pipeline=off
      settings: xl_area=[0, 0, 0, 0, 0, 0, 0]
  Convert4 : xbsIndex_r3/Convert  Orientation=left  arith_type=Boolean  n_bits=8  bin_pt=6  quantization=Truncate  overflow=Wrap  latency=0  explicit_period=off  period=1  dbl_ovrd=off  show_param=off  inserted_by_tool=off  pipeline=off
      settings: xl_area=[0, 0, 0, 0, 0, 0, 0]
  Gateway Out{1..20,29..35} (27 alike) : xbsIndex_r3/Gateway Out  output_type=Double  nbits=8  bin_pt=6  arith_type=Boolean  quantization=Truncate  overflow=Wrap  hdl_port=on  timing_constraint=None  locs_specified=off  LOCs={}  needs_fixed_name=off  show_param=off
      settings: xl_area=[0, 0, 0, 0, 0, 0, 0]
  Inverter : xbsIndex_r3/Inverter  Orientation=left  latency=0  explicit_period=off  period=1  en=off  dbl_ovrd=off  show_param=off
      settings: xl_area=[0, 0, 0, 0, 0, 0, 0]
  Inverter1 : xbsIndex_r3/Inverter  Orientation=left  latency=0  explicit_period=off  period=1  en=off  dbl_ovrd=off  show_param=off
      settings: xl_area=[0, 0, 0, 0, 0, 0, 0]
  Inverter4 : xbsIndex_r3/Inverter  latency=0  explicit_period=off  period=1  en=off  dbl_ovrd=off  show_param=off
      settings: xl_area=[0, 0, 0, 0, 0, 0, 0]
  Inverter5 : xbsIndex_r3/Inverter  latency=0  explicit_period=off  period=1  en=off  dbl_ovrd=off  show_param=off
      settings: xl_area=[0, 0, 0, 0, 0, 0, 0]
  Mux{,1..5} (6 alike) : xbsIndex_r3/Mux  inputs=2  precision=Full  arith_type="Signed  (2's comp)"  n_bits=8  bin_pt=2  quantization=Truncate  overflow=Wrap  latency=0  explicit_period=on  period=1  en=off  dbl_ovrd=off  show_param=off  mux_type=off  use_rpm=off  gen_core=off
      settings: xl_area=[0, 0, 0, 0, 0, 0, 0]
  Register : xbsIndex_r3/Register  init=0  reg_only_valid=off  explicit_period=on  period=1  rst=on  en=on  out_en=off  dbl_ovrd=off  show_param=off
      settings: xl_area=[0, 0, 0, 0, 0, 0, 0]
  Slice : xbsIndex_r3/Slice  mode=Lower Bit Location + Width  nbits=1  bit1=0  base1=MSB of Input  bit0=0  base0=LSB of Input  boolean_output=on  explicit_period=off  period=1  dbl_ovrd=off
  Slice{1..3,5,7} (5 alike) : xbsIndex_r3/Slice  mode=Upper Bit Location + Width  nbits=1  bit1=0  base1=MSB of Input  bit0=0  base0=LSB of Input  boolean_output=off  explicit_period=off  period=1  dbl_ovrd=off
  Slice4 : xbsIndex_r3/Slice  mode=Lower Bit Location + Width  nbits=64  bit1=0  base1=MSB of Input  bit0=0  base0=LSB of Input  boolean_output=off  explicit_period=off  period=1  dbl_ovrd=off
  Slice6 : xbsIndex_r3/Slice  Orientation=up  mode=Lower Bit Location + Width  nbits=64  bit1=0  base1=MSB of Input  bit0=0  base0=LSB of Input  boolean_output=off  explicit_period=off  period=1  dbl_ovrd=off
  d_in_0_debug : Scope  NumInputPorts=4
      settings: YMin=100~0~0~-1  YMax=1400~1~1~1  SaveName=ScopeData2
  d_out_1_debug : Scope  NumInputPorts=4
      settings: YMin=100~0~0~-1  YMax=1000~1~1~1  SaveName=ScopeData3
  dest_ip_sel : xbsIndex_r3/Mux  inputs=2  precision=Full  arith_type="Signed  (2's comp)"  n_bits=8  bin_pt=2  quantization=Truncate  overflow=Wrap  latency=0  explicit_period=off  period=1  en=off  dbl_ovrd=off  show_param=off  mux_type=off  use_rpm=off  gen_core=off
      settings: xl_area=[0, 0, 0, 0, 0, 0, 0]
  dout_and_eof_sel : xbsIndex_r3/Mux  inputs=2  precision=Full  arith_type="Signed  (2's comp)"  n_bits=8  bin_pt=2  quantization=Truncate  overflow=Wrap  latency=0  explicit_period=off  period=1  en=off  dbl_ovrd=off  show_param=off  mux_type=off  use_rpm=off  gen_core=off
      settings: xl_area=[0, 0, 0, 0, 0, 0, 0]
  enable_rd_from_1 : xbsIndex_r3/Logical  logical_function=AND  inputs=2  precision=Full  arith_type=Unsigned  n_bits=8  bin_pt=2  align_bp=on  latency=0  explicit_period=off  period=1  en=off  dbl_ovrd=off  show_param=off
      settings: xl_area=[0, 0, 0, 0, 0, 0, 0]
  enable_rd_from_2 : xbsIndex_r3/Logical  logical_function=AND  inputs=2  precision=Full  arith_type=Unsigned  n_bits=8  bin_pt=2  align_bp=on  latency=0  explicit_period=off  period=1  en=off  dbl_ovrd=off  show_param=off
      settings: xl_area=[0, 0, 0, 0, 0, 0, 0]
  enable_rd_from_3 : xbsIndex_r3/Logical  logical_function=AND  inputs=2  precision=Full  arith_type=Unsigned  n_bits=8  bin_pt=2  align_bp=on  latency=0  explicit_period=off  period=1  en=off  dbl_ovrd=off  show_param=off
      settings: xl_area=[0, 0, 0, 0, 0, 0, 0]
  fifo_empty : xbsIndex_r3/Logical  logical_function=AND  inputs=4  precision=Full  arith_type=Unsigned  n_bits=8  bin_pt=2  align_bp=on  latency=0  explicit_period=off  period=1  en=off  dbl_ovrd=off  show_param=off
      settings: xl_area=[0, 0, 0, 0, 0, 0, 0]
  fifo_full : xbsIndex_r3/Logical  logical_function=OR  inputs=4  precision=Full  arith_type=Unsigned  n_bits=8  bin_pt=2  align_bp=on  latency=0  explicit_period=off  period=1  en=off  dbl_ovrd=off  show_param=off
      settings: xl_area=[0, 0, 0, 0, 0, 0, 0]
  fifo_full1 : xbsIndex_r3/Logical  logical_function=OR  inputs=3  precision=Full  arith_type=Unsigned  n_bits=8  bin_pt=2  align_bp=on  latency=0  explicit_period=off  period=1  en=off  dbl_ovrd=off  show_param=off
      settings: xl_area=[0, 0, 0, 0, 0, 0, 0]
  flush : xps_library/software register  Tag=xps:sw_reg  io_dir=From Processor  arith_type=Unsigned  bitwidth=32  bin_pt=0  sample_period=1  gw_name=test_dram_sim_mux_pack_it1_flush_user_data_out
  fwft_fifo_data : Subsystem
  fwft_fifo_ip_addr : Subsystem
  in0_data : Subsystem  mask{depth_bits=ceil(log2(max(max_packet_size_0,max_packet_size_1))) +1}
      mask prompts: depth_bits "Fifo Depth (2^?):"
      mask help: A rollback fifo behaves as a normal fifo, except that data which are written in have to be "committed" before they become available for readout. Moreover, any data which are written in and have not been committed can be "discarded", and will never be made available for readout.
  in0_ip_addr : Subsystem  mask{depth_bits=ceil(log2(ceil((max_packet_size_1 / min_packet_size_0))))+1}
      mask prompts: depth_bits "Fifo Depth (2^?):"
      mask help: A rollback fifo behaves as a normal fifo, except that data which are written in have to be "committed" before they become available for readout. Moreover, any data which are written in and have not been committed can be "discarded", and will never be made available for readout.
  in1_data : Subsystem  mask{depth_bits=ceil(log2(max(max_packet_size_0,max_packet_size_1))) +1}
      mask prompts: depth_bits "Fifo Depth (2^?):"
      mask help: A rollback fifo behaves as a normal fifo, except that data which are written in have to be "committed" before they become available for readout. Moreover, any data which are written in and have not been committed can be "discarded", and will never be made available for readout.
  in1_ip_addr : Subsystem  mask{depth_bits=ceil(log2(ceil((max_packet_size_0 / min_packet_size_1))))+1}
      mask prompts: depth_bits "Fifo Depth (2^?):"
      mask help: A rollback fifo behaves as a normal fifo, except that data which are written in have to be "committed" before they become available for readout. Moreover, any data which are written in and have not been committed can be "discarded", and will never be made available for readout.
  mux_buffer_full : Scope  NumInputPorts=6
      settings: TimeRange=1500  YMin=100~0~0~-1~-5~-5  YMax=1400~1~1~1~5~5  SaveName=ScopeData11
  mux_debug : Scope  NumInputPorts=9
      settings: YMin=0~0~0~0~0~0~0~-5~-5  YMax=1~1~1~1~1~1~1~5~5  SaveName=ScopeData10
  mux_out_debug : Scope  NumInputPorts=4
      settings: YMin=100~0~0~-1  YMax=1400~1~1~1  SaveName=ScopeData5
  sel_1 : xbsIndex_r3/Inverter  Orientation=up  latency=0  explicit_period=off  period=1  en=off  dbl_ovrd=off  show_param=off
      settings: xl_area=[0, 0, 0, 0, 0, 0, 0]
  we_sel : xbsIndex_r3/Mux  inputs=2  precision=Full  arith_type="Signed  (2's comp)"  n_bits=8  bin_pt=2  quantization=Truncate  overflow=Wrap  latency=0  explicit_period=off  period=1  en=off  dbl_ovrd=off  show_param=off  mux_type=off  use_rpm=off  gen_core=off
      settings: xl_area=[0, 0, 0, 0, 0, 0, 0]
  data : Outport
  valid : Outport  Port=2
  ip_addr : Outport  Port=3
  eof : Outport  Port=4
  discard : Outport  Port=5
  buffer_overflow : Outport  Port=6
  buffer_empty : Outport  Port=7
  ack_0 : Outport  Port=8
  ack_1 : Outport  Port=9
  wires:
  in0_ip_addr/1(dout) -> dest_ip_sel/2
  in0_data/2(valid) -> we_sel/2, Gateway Out34/1
  in0_data/1(dout) -> Slice1/1, dout_and_eof_sel/2
  discard_0/1 -> in0_data/4(discard), in0_ip_addr/4(discard)
  in0_data/5(empty) -> fifo_empty/2, Gateway Out13/1, Inverter1/1
  Concat/1 -> in0_data/1(din)
  Slice1/1 -> Convert/1
  Convert/1 -> Gateway Out31/1, 0_fin_AND_1_not_empty/1, Mux1/2
  in0_data/4(full) -> Inverter4/1, fifo_full/2, Gateway Out18/1
  Inverter4/1 -> enable_rd_from_2/2
  in0_ip_addr/4(full) -> fifo_full/1, Gateway Out17/1
  in0_ip_addr/5(empty) -> fifo_empty/1
  in1_ip_addr/1(dout) -> dest_ip_sel/3
  in1_data/2(valid) -> Gateway Out6/1, Gateway Out35/1, we_sel/3
  in1_data/1(dout) -> Slice3/1, dout_and_eof_sel/3, Gateway Out8/1
  discard_1/1 -> in1_ip_addr/4(discard), in1_data/4(discard)
  in1_data/5(empty) -> fifo_empty/4, Inverter/1, Gateway Out14/1
  Concat1/1 -> in1_data/1(din)
  Slice3/1 -> Convert1/1
  Convert1/1 -> Gateway Out33/1, 1_fin_AND_0_valid/2, Mux3/2
  in1_data/4(full) -> Inverter5/1, fifo_full/4, Gateway Out16/1
  Inverter5/1 -> enable_rd_from_3/2
  enable_rd_from_2/1 -> in0_ip_addr/3(commit), in0_ip_addr/2(we)
  in1_ip_addr/5(empty) -> fifo_empty/3
  enable_rd_from_3/1 -> in1_ip_addr/3(commit), in1_ip_addr/2(we)
  in1_ip_addr/4(full) -> fifo_full/3, Gateway Out15/1
  Register/1 -> sel_1/1, Gateway Out32/1, Mux2/2, dout_and_eof_sel/1, we_sel/1, dest_ip_sel/1, Gateway Out4/1
  Constant12/1 -> Register/1
  Gateway Out32/1 -> mux_debug/1
  Gateway Out29/1 -> mux_debug/2
  Gateway Out30/1 -> mux_debug/3
  Gateway Out31/1 -> mux_debug/4
  Gateway Out33/1 -> mux_debug/5
  Gateway Out34/1 -> mux_debug/6
  Gateway Out35/1 -> mux_debug/7
  d_in_0/1 -> Concat/2, Gateway Out1/1
  valid_0/1 -> Gateway Out2/1, in0_data/2(we)
  dest_ip_0/1 -> in0_ip_addr/1(din)
  eof_0/1 -> enable_rd_from_2/1, Concat/1, Gateway Out3/1, in0_data/3(commit)
  d_in_1/1 -> Concat1/2, Gateway Out5/1
  valid_1/1 -> in1_data/2(we)
  dest_ip_1/1 -> in1_ip_addr/1(din)
  eof_1/1 -> enable_rd_from_3/1, Concat1/1, Gateway Out7/1, in1_data/3(commit)
  in0_data/3(wr_ack) -> ack_0/1
  in1_data/3(wr_ack) -> ack_1/1
  Convert2/1 -> valid/1
  Gateway Out4/1 -> d_in_0_debug/1
  Gateway Out1/1 -> d_in_0_debug/2
  Gateway Out2/1 -> d_in_0_debug/3
  Gateway Out3/1 -> d_in_0_debug/4
  Gateway Out8/1 -> d_out_1_debug/1
  Gateway Out5/1 -> d_out_1_debug/2
  Gateway Out6/1 -> d_out_1_debug/3
  Gateway Out7/1 -> d_out_1_debug/4
  0_fin_AND_1_not_empty/1 -> Convert3/1
  1_fin_AND_0_valid/1 -> Convert4/1
  Convert3/1 -> Register/3, Gateway Out30/1
  Convert4/1 -> Register/2, Gateway Out29/1
  Constant13/1 -> discard/1
  Slice2/1 -> Convert5/1
  dout_and_eof_sel/1 -> Slice5/1, fwft_fifo_data/1(din), Slice7/1, Slice6/1
  Convert5/1 -> eof/1, enable_rd_from_1/2
  Slice4/1 -> data/1
  fwft_fifo_data/2(valid) -> Convert2/1
  we_sel/1 -> fwft_fifo_data/2(we), Gateway Out9/1
  rd_ack/1 -> enable_rd_from_1/1, Mux4/2
  dest_ip_sel/1 -> Gateway Out10/1, fwft_fifo_ip_addr/1(din)
  Slice5/1 -> Convert6/1
  Convert6/1 -> fwft_fifo_ip_addr/2(we)
  fwft_fifo_ip_addr/1(dout) -> ip_addr/1
  Gateway Out12/1 -> mux_out_debug/1
  Gateway Out9/1 -> mux_out_debug/2
  Gateway Out10/1 -> mux_out_debug/3
  Gateway Out11/1 -> mux_out_debug/4
  fwft_fifo_data/1(dout) -> Slice4/1, Slice2/1
  fifo_full1/1 -> buffer_overflow/1
  fwft_fifo_data/3(overflow) -> fifo_full1/1, Gateway Out19/1
  fwft_fifo_ip_addr/3(overflow) -> fifo_full1/2, Gateway Out20/1
  fifo_full/1 -> fifo_full1/3
  fifo_empty/1 -> buffer_empty/1
  Gateway Out13/1 -> mux_debug/8
  Gateway Out14/1 -> mux_debug/9
  Slice6/1 -> Gateway Out12/1
  Slice7/1 -> Gateway Out11/1
  Gateway Out17/1 -> mux_buffer_full/1
  Gateway Out18/1 -> mux_buffer_full/2
  Gateway Out15/1 -> mux_buffer_full/3
  Gateway Out16/1 -> mux_buffer_full/4
  Gateway Out19/1 -> mux_buffer_full/5
  Gateway Out20/1 -> mux_buffer_full/6
  Constant/1 -> flush/1
  flush/1 -> Slice/1
  Mux/1 -> in0_data/5(rd_ack)
  sel_1/1 -> Mux/2
  Constant1/1 -> Mux/3
  Constant2/1 -> Mux1/3
  Mux1/1 -> in0_ip_addr/5(rd_ack)
  Constant3/1 -> Mux2/3
  Mux2/1 -> in1_data/5(rd_ack)
  Constant4/1 -> Mux3/3
  Mux3/1 -> in1_ip_addr/5(rd_ack)
  [flush_buffers] -> Mux/1
  [flush_buffers] -> Mux1/1
  [flush_buffers] -> Mux2/1
  [flush_buffers] -> Mux3/1
  Constant5/1 -> Mux4/3
  [flush_buffers] -> Mux4/1
  Mux4/1 -> fwft_fifo_data/3(ack)
  Constant6/1 -> Mux5/3
  [flush_buffers] -> Mux5/1
  Mux5/1 -> fwft_fifo_ip_addr/3(ack)
  enable_rd_from_1/1 -> Mux5/2
  Slice/1 -> [flush_buffers]
  Inverter/1 -> 0_fin_AND_1_not_empty/2
  Inverter1/1 -> 1_fin_AND_0_valid/1
